simulink subsystem "Clark"  (R2023b)
settings: Solver=VariableStepAuto  StartTime=0.0  StopTime=10.0  RelTol=1e-3
settings Model: Creator=rainy  LastModifiedBy=rainy

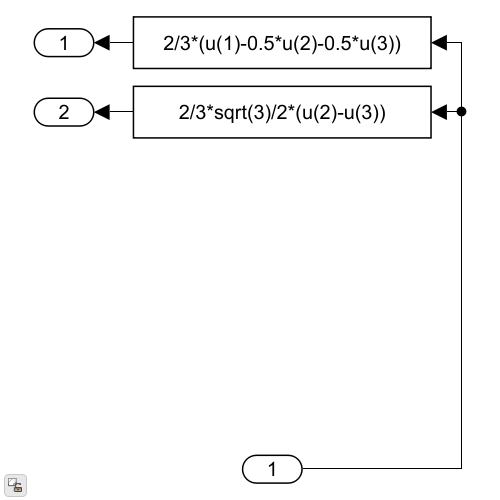
[thumbnail: Simulink's stored preview of the top-level diagram]
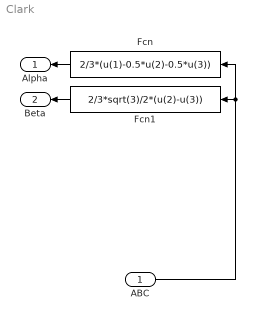
== system Clark ==
  ABC : Inport
  Fcn : Fcn  Expr=2/3*(u(1)-0.5*u(2)-0.5*u(3))
  Fcn1 : Fcn  Expr=2/3*sqrt(3)/2*(u(2)-u(3))
  Alpha : Outport
  Beta : Outport  Port=2
  wires:
  ABC/1 -> Fcn/1, Fcn1/1
  Fcn1/1 -> Beta/1
  Fcn/1 -> Alpha/1
